simulink model "SunsensorActuatorsDrag"  (R2021b)
settings: Solver=FixedStepAuto  StartTime=0.0  StopTime=T  FixedStep=0.1  RelTol=1e-3
values from neighbouring files (symbols this model uses):
  a = 1/( 2/norm(r0) - dot(v0,v0)/mu_E )    [Excercise1_2223.m]    (also in Excercise2_2223.m; Lab08_script.m = 42164; Lab7_script.m = 16733.65; Lab7_scriptscalar.m = 16733.65)
  A0 = eye(3)    [Lab08_script.m]    (also in Lab7_script.m; Lab7_scriptscalar.m; Lab_GG.m)
  alpha = deg2rad(11.5)    [Lab08_script.m]
  Area_mb = diag([A1 A2 A3 A4 A5 A6])    [Lab08_script.m]    (also in Lab7_script.m)
  Area_sp = diag([A7 A8 A9 A10])    [Lab08_script.m]    (also in Lab7_script.m)
  around_boresight = deg2rad(dms2degrees([0,0,around_boresight]))    [Lab08_script.m]
  cross_boresight = deg2rad(dms2degrees([0,0,cross_boresight]))    [Lab08_script.m]
  e = horizonsresults(:,2)    [Ex3-5.m]    (also in Excercise1_2223.m = 1/mu_E*cross(v,h)-r./vecnorm(r,2,2); Lab08_script.m = 0; Lab7_script.m = 0.1976; Lab7_scriptscalar.m = 0.1976)
  epsilon = (vecnorm(v,2,2)).^2/2-mu_E./vecnorm(r,2,2)    [Excercise1_2223.m]    (also in Lab08_script.m = deg2rad(23.45); Lab7_script.m = deg2rad(23.45); Lab7_scriptscalar.m = deg2rad(23.45))
  H0 = ( g1_0^2 + g1_1^2 + h1_1^2 )^(1/2)    (= 3.0115258674e-05)    [Lab08_script.m]
  I = [Ix 0 0; 0 Iy 0; 0 0 Iz]    [Lab08_script.m]    (also in Lab7_script.m; Lab7_scriptscalar.m; Lab_GG.m)
  i = horizonsresults(:,3)    [Ex3-5.m]    (also in Lab08_script.m = deg2rad(0); Lab7_script.m = deg2rad(60); Lab7_scriptscalar.m = deg2rad(60); ex3_Lambert.m = kep_arr_M(3))
  I_inv = inv(I)    [Lab08_script.m]    (also in Lab7_script.m; Lab7_scriptscalar.m; Lab_GG.m)
  i_matrix = [1 0 0; 0 cos(i) sin(i); 0 -sin(i) cos(i)]    [Lab08_script.m]
  m = [0.01; 0.05; 0.01]    [Lab08_script.m]
  mu_E = astroConstants(13)    [Chapter3.m]    (also in Ex3-5.m; Excercise1_2223.m; Excercise2_2223.m; Lab08_script.m)
  n = 10    [Chapter3.m]    (also in Lab08_script.m = sqrt(mu_E/(a^3)); Lab7_script.m = sqrt(mu_E/(a^3)); Lab7_scriptscalar.m = sqrt(mu_E/(a^3)); Lab_GG.m = sqrt(mu_E/( R_E+r_orbit)^3))
  n3 = [0;0;1]    [Lab08_script.m]    (also in Lab7_script.m; Lab7_scriptscalar.m)
  N_b_mb = [n1'; n2'; n3'; n4'; n5'; n6']    [Lab08_script.m]    (also in Lab7_script.m)
  N_b_sp = [n7'; n8'; n9'; n10']    [Lab08_script.m]    (also in Lab7_script.m)
  n_sun = 2*pi/T_sun    (= 1.99238499086e-07)    [Lab08_script.m]    (also in Lab7_script.m; Lab7_scriptscalar.m)
  P = Fe/c    (= 4.52666666667e-06)    [Lab08_script.m]    (also in Lab7_script.m; Lab7_scriptscalar.m)
  R_E = astroConstants(23)    [Lab08_script.m]    (also in Lab7_script.m; Lab7_scriptscalar.m; Lab_GG.m)
  r_mb = [base/2 0 0; 0 base/2 0; 0 0 height/2; -base/2 0 0; 0 -base/2 0; 0 0 -height/2]    [Lab08_script.m]
  r_sp = [0 length_p1/2+base/2 0; 0 length_p1/2+base/2 0; 0 -length_p2/2-base/2 0; 0 -length_p2/2-base/2 0]    [Lab08_script.m]
  rho_s_mb = 0.5    [Lab08_script.m]    (also in Lab7_script.m; Lab7_scriptscalar.m)
  rho_s_sp = 0.1    [Lab08_script.m]    (also in Lab7_script.m; Lab7_scriptscalar.m)
  Rs = astroConstants(2)    [Lab08_script.m]    (also in Lab7_script.m; Lab7_scriptscalar.m)
  theta0 = deg2rad(0)    [Lab08_script.m]    (also in Lab7_script.m = deg2rad(230); Lab7_scriptscalar.m = deg2rad(230))
  unit = [1 0 0]'    [Lab08_script.m]    (also in Lab_GG.m)
  v1 = [Y1(:,4) Y1(:,5) Y1(:,6)]    [Excercise2_2223.m]    (also in Lab08_script.m = [0 1 -1]'; Lab7_script.m = [0 1 -1]'; Lab7_scriptscalar.m = [0 1 -1]'; Lab_GG.m = [0 1 -1]')
  v2 = [Y2(:,4) Y2(:,5) Y2(:,6)]    [Excercise2_2223.m]    (also in Lab08_script.m = [-1 0 1]'; Lab7_script.m = [-1 0 1]'; Lab7_scriptscalar.m = [-1 0 1]'; Lab_GG.m = [-1 0 1]')
  v3 = [1 -1 0]'    [Lab08_script.m]    (also in Lab7_script.m; Lab7_scriptscalar.m; Lab_GG.m)
  w_0 = [wx_0 wy_0 wz_0]'    [Lab08_script.m]    (also in Lab7_script.m; Lab7_scriptscalar.m; Lab_GG.m)
  w_E = deg2rad(15.04/3600)    [Ex3-5.m]    (also in Lab08_script.m = deg2rad(15.04)/3600)
  wy_0 = 1e-06    [Lab08_script.m]    (also in Lab7_script.m; Lab7_scriptscalar.m; Lab_GG.m = 0)
undefined symbols (not defined in the file or in its folder): A_vect, Cd, h_N_target, L, m_N_unit, N_B_Matrix, weight
libraries: matrix_library x15, vrlib x13, dspmtrx3 x2, sharedutil x2, simulink_extras x1
(part 1 of 2)
settings Model: Creator=sferl  LastModifiedBy=Giovanni

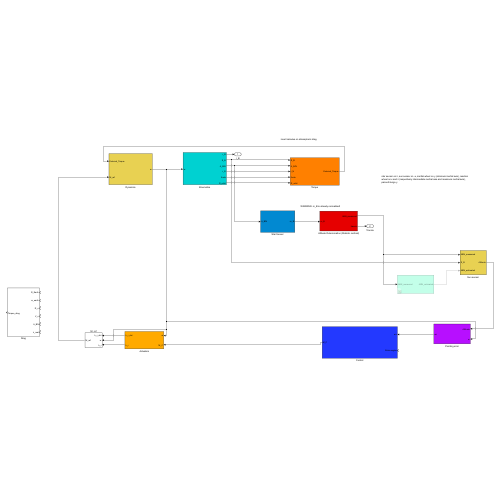
[thumbnail: Simulink's stored preview of the top-level diagram]
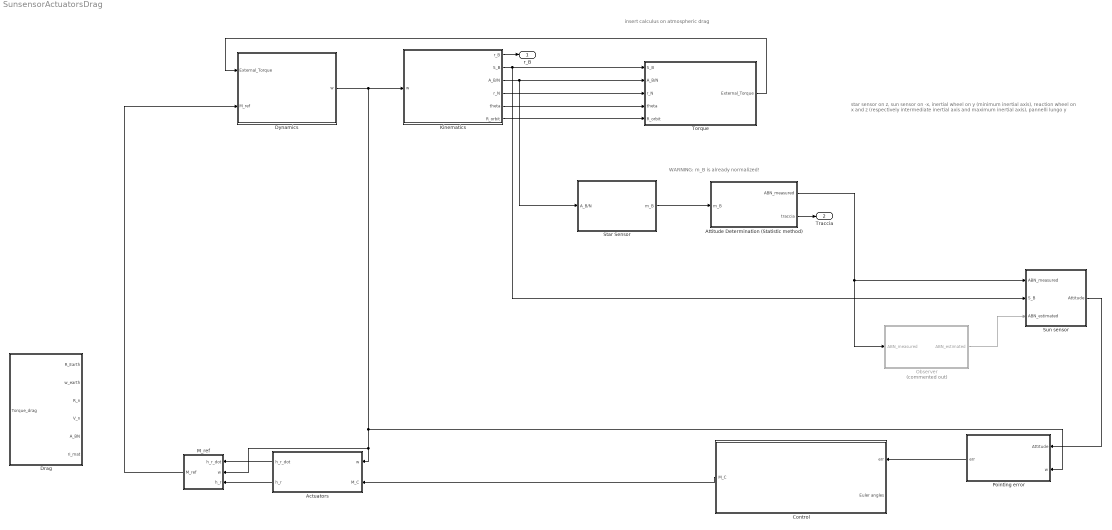
== system SunsensorActuatorsDrag ==
  note: insert calculus on atmospheric drag
  note: star sensor on z, sun sensor on -x, inertial wheel on y (minimum inertial axis), reaction wheel on x and z (respectively intermediate inertial axis and maximum inertial axis), pannelli lungo y
  note: WARNING: m_B is already normalized!
  Actuators : Subsystem
  Attitude Determination (Statistic method) : Subsystem
  Control : Subsystem
  Drag : Subsystem
  Dynamics : Subsystem
  Kinematics : Subsystem
  M_ref : Subsystem
  Observer : Subsystem  Commented=on
  Pointing error : Subsystem
  Star Sensor : Subsystem
  Sun sensor : Subsystem
  Torque : Subsystem
  r_B : Outport
  Traccia : Outport  Port=2
  wires:
  Kinematics/1(r_B) -> r_B/1
  Kinematics/3(A_B/N) -> Star Sensor/1(A_B/N), Torque/2(A_B/N)
  Star Sensor/1(m_B) -> Attitude Determination (Statistic method)/1(m_B)
  Kinematics/2(S_B) -> Sun sensor/2(S_B), Torque/1(S_B)
  Kinematics/4(r_N) -> Torque/3(r_N)
  Kinematics/5(theta) -> Torque/4(theta)
  Kinematics/6(R_orbit) -> Torque/5(R_orbit)
  Torque/1(External_Torque) -> Dynamics/1(External_Torque)
  Dynamics/1(w) -> Actuators/1(w), M_ref/2(w), Pointing error/2(w), Kinematics/1(w)
  Attitude Determination (Statistic method)/2(traccia) -> Traccia/1
  Pointing error/1(err) -> Control/1(err)
  Sun sensor/1(Attitude) -> Pointing error/1(Attitude)
  Attitude Determination (Statistic method)/1(ABN_measured) -> Sun sensor/1(ABN_measured), Observer/1(ABN_measured)
  Observer/1(ABN_estimated) -> Sun sensor/3(ABN_estimated)
  Control/1(M_C) -> Actuators/2(M_C)
  Actuators/1(h_r_dot) -> M_ref/1(h_r_dot)
  Actuators/2(h_r) -> M_ref/3(h_r)
  M_ref/1(M_ref) -> Dynamics/2(M_ref)

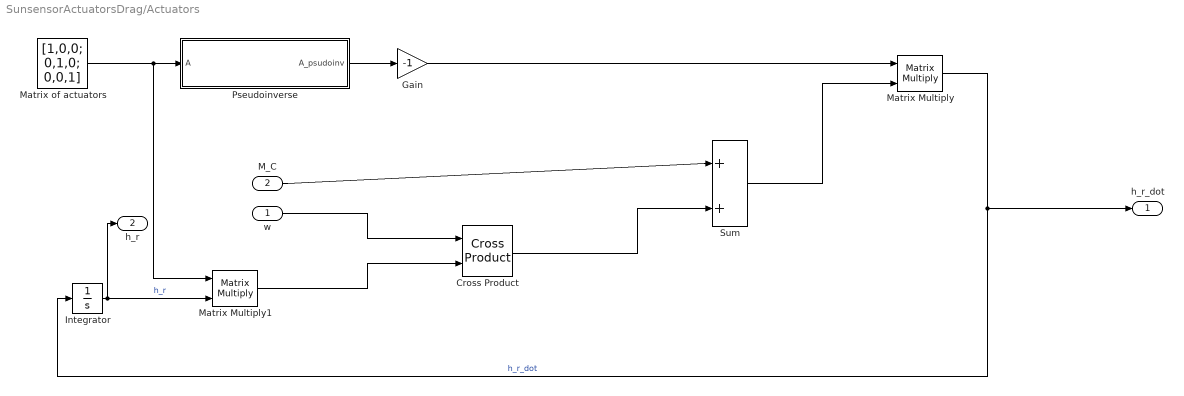
== system SunsensorActuatorsDrag/Actuators ==
  w : Inport
  M_C : Inport  Port=2
  Cross Product : matrix_library/Cross Product
  Gain : Gain  Gain=-1
  Integrator : Integrator  InitialCondition=[0; wy_0; 0]
  Matrix Multiply : Product  Multiplication=Matrix(*)
  Matrix Multiply1 : Product  Multiplication=Matrix(*)
  Matrix of actuators : Constant  Value=[1,0,0; 0,1,0; 0,0,1]
  Pseudoinverse : MATLAB Function  TreatAsAtomicUnit=on
  Sum : Sum  Inputs=|++
  h_r_dot : Outport
  h_r : Outport  Port=2
  wires:
  Matrix of actuators/1 -> Matrix Multiply1/1, Pseudoinverse/1(A)
  Pseudoinverse/1(A_psudoinv) -> Gain/1
  Gain/1 -> Matrix Multiply/1
  M_C/1 -> Sum/1
  w/1 -> Cross Product/1
  Matrix Multiply/1 -> h_r_dot/1, Integrator/1  "h_r_dot"
  Integrator/1 -> h_r/1, Matrix Multiply1/2  "h_r"
  Matrix Multiply1/1 -> Cross Product/2
  Cross Product/1 -> Sum/2
  Sum/1 -> Matrix Multiply/2

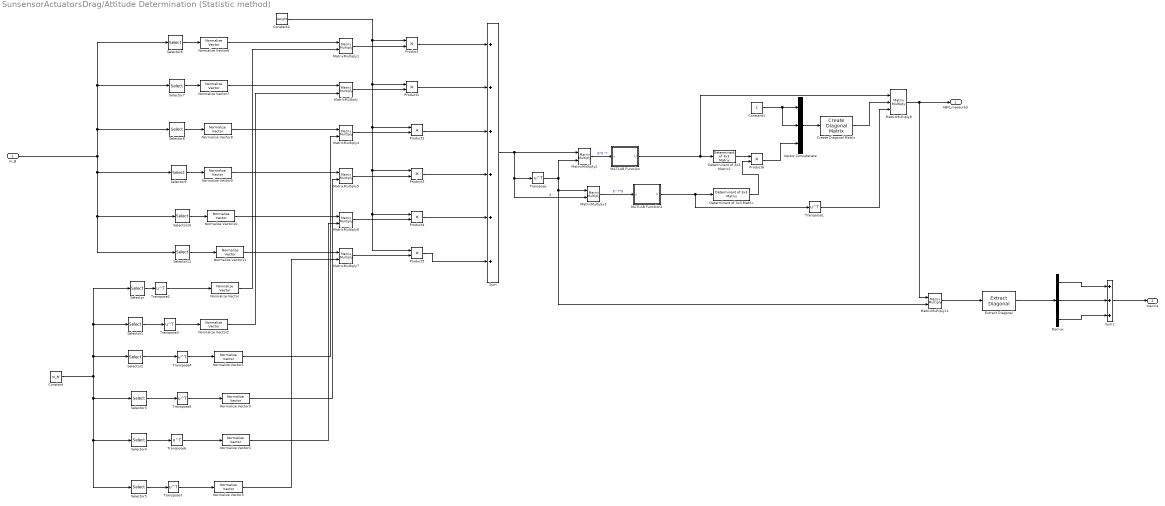
== system SunsensorActuatorsDrag/Attitude Determination (Statistic method) ==
  m_B : Inport
  Constant : Constant  Value=m_N'
  Constant1 : Constant
  Constant2 : Constant  Value=weight
  Create Diagonal Matrix : dspmtrx3/Create Diagonal Matrix
  Demux : Demux  Outputs=3
  Determinant of 3x3 Matrix : sharedutil/Determinant of 3x3 Matrix  aMode=aMode
  Determinant of 3x3 Matrix1 : sharedutil/Determinant of 3x3 Matrix  aMode=aMode
  Extract Diagonal : dspmtrx3/Extract Diagonal
  MATLAB Function : MATLAB Function  TreatAsAtomicUnit=on
  MATLAB Function1 : MATLAB Function  TreatAsAtomicUnit=on
  MatrixMultiply{,1..7,11} (9 alike) : Product  Multiplication=Matrix(*)
  MatrixMultiply8 : Product  Inputs=3  Multiplication=Matrix(*)
  Normalize Vector{,1..11} (12 alike) : vrlib/Utilities/Normalize Vector  maxzero=0
  Product{,1..6} (7 alike) : Product
  Selector : Selector  NumberOfDimensions=2  InputPortWidth=3  IndexOptions=Starting index (dialog),Starting index (dialog)  Indices=1,1  OutputSizes=3,1
  Selector1 : Selector  NumberOfDimensions=2  InputPortWidth=3  IndexOptions=Starting index (dialog),Starting index (dialog)  Indices=1,2  OutputSizes=3,1
  Selector10 : Selector  NumberOfDimensions=2  InputPortWidth=3  IndexOptions=Starting index (dialog),Starting index (dialog)  Indices=1,5  OutputSizes=3,1
  Selector11 : Selector  NumberOfDimensions=2  InputPortWidth=3  IndexOptions=Starting index (dialog),Starting index (dialog)  Indices=1,6  OutputSizes=3,1
  Selector2 : Selector  NumberOfDimensions=2  InputPortWidth=3  IndexOptions=Starting index (dialog),Starting index (dialog)  Indices=1,3  OutputSizes=3,1
  Selector3 : Selector  NumberOfDimensions=2  InputPortWidth=3  IndexOptions=Starting index (dialog),Starting index (dialog)  Indices=1,4  OutputSizes=3,1
  Selector4 : Selector  NumberOfDimensions=2  InputPortWidth=3  IndexOptions=Starting index (dialog),Starting index (dialog)  Indices=1,5  OutputSizes=3,1
  Selector5 : Selector  NumberOfDimensions=2  InputPortWidth=3  IndexOptions=Starting index (dialog),Starting index (dialog)  Indices=1,6  OutputSizes=3,1
  Selector6 : Selector  NumberOfDimensions=2  InputPortWidth=3  IndexOptions=Starting index (dialog),Starting index (dialog)  Indices=1,1  OutputSizes=3,1
  Selector7 : Selector  NumberOfDimensions=2  InputPortWidth=3  IndexOptions=Starting index (dialog),Starting index (dialog)  Indices=1,2  OutputSizes=3,1
  Selector8 : Selector  NumberOfDimensions=2  InputPortWidth=3  IndexOptions=Starting index (dialog),Starting index (dialog)  Indices=1,3  OutputSizes=3,1
  Selector9 : Selector  NumberOfDimensions=2  InputPortWidth=3  IndexOptions=Starting index (dialog),Starting index (dialog)  Indices=1,4  OutputSizes=3,1
  Sum : Sum  Inputs=++++++
  Sum1 : Sum  Inputs=+++
  Transpose{,1..7} (8 alike) : Math  Operator=transpose  SaturateOnIntegerOverflow=on
  Vector Concatenate : Concatenate  NumInputs=3
  ABN_measured : Outport
  traccia : Outport  Port=2
  wires:
  Transpose/1 -> MatrixMultiply11/2, MatrixMultiply3/1, MatrixMultiply2/2
  Constant2/1 -> Product3/1, Product4/1, Product5/1, Product2/1, Product1/1, Product/1
  Product2/1 -> Sum/3
  MatrixMultiply/1 -> Product1/2
  Product1/1 -> Sum/2
  MatrixMultiply7/1 -> Product5/2
  Sum/1 -> MatrixMultiply3/2, Transpose/1, MatrixMultiply2/1  "B"
  MatrixMultiply2/1 -> MATLAB Function/1(u)  "B*B^T"
  Product5/1 -> Sum/6
  MatrixMultiply5/1 -> Product3/2
  Product4/1 -> Sum/5
  Product/1 -> Sum/1
  MatrixMultiply4/1 -> Product2/2
  MatrixMultiply1/1 -> Product/2
  Product3/1 -> Sum/4
  MatrixMultiply6/1 -> Product4/2
  Selector1/1 -> Transpose3/1
  Selector3/1 -> Transpose5/1
  Selector4/1 -> Transpose6/1
  Constant/1 -> Selector3/1, Selector4/1, Selector5/1, Selector/1, Selector1/1, Selector2/1
  Selector2/1 -> Transpose4/1
  Selector5/1 -> Transpose7/1
  m_B/1 -> Selector6/1, Selector7/1, Selector8/1, Selector11/1, Selector10/1, Selector9/1
  Determinant of 3x3 Matrix1/1 -> Product6/1
  Determinant of 3x3 Matrix/1 -> Product6/2
  Constant1/1 -> Vector Concatenate/2, Vector Concatenate/1
  Product6/1 -> Vector Concatenate/3
  Vector Concatenate/1 -> Create Diagonal Matrix/1
  Create Diagonal Matrix/1 -> MatrixMultiply8/2
  MATLAB Function/1(U) -> MatrixMultiply8/1, Determinant of 3x3 Matrix1/1
  Transpose1/1 -> MatrixMultiply8/3
  MatrixMultiply8/1 -> MatrixMultiply11/1, ABN_measured/1
  MatrixMultiply3/1 -> MATLAB Function1/1(u)  "B^T*B"
  MATLAB Function1/1(V) -> Transpose1/1, Determinant of 3x3 Matrix/1
  MatrixMultiply11/1 -> Extract Diagonal/1
  Extract Diagonal/1 -> Demux/1
  Demux/1 -> Sum1/1
  Demux/2 -> Sum1/2
  Demux/3 -> Sum1/3
  Sum1/1 -> traccia/1
  Selector6/1 -> Normalize Vector6/1
  Selector7/1 -> Normalize Vector7/1
  Selector8/1 -> Normalize Vector8/1
  Selector9/1 -> Normalize Vector9/1
  Selector10/1 -> Normalize Vector10/1
  Selector11/1 -> Normalize Vector11/1
  Selector/1 -> Transpose2/1
  Transpose3/1 -> Normalize Vector2/1
  Transpose2/1 -> Normalize Vector/1
  Transpose4/1 -> Normalize Vector1/1
  Transpose5/1 -> Normalize Vector3/1
  Transpose6/1 -> Normalize Vector4/1
  Transpose7/1 -> Normalize Vector5/1
  Normalize Vector/1 -> MatrixMultiply1/2
  Normalize Vector2/1 -> MatrixMultiply/2
  Normalize Vector1/1 -> MatrixMultiply4/2
  Normalize Vector3/1 -> MatrixMultiply5/2
  Normalize Vector4/1 -> MatrixMultiply6/2
  Normalize Vector5/1 -> MatrixMultiply7/2
  Normalize Vector6/1 -> MatrixMultiply1/1
  Normalize Vector7/1 -> MatrixMultiply/1
  Normalize Vector8/1 -> MatrixMultiply4/1
  Normalize Vector9/1 -> MatrixMultiply5/1
  Normalize Vector10/1 -> MatrixMultiply6/1
  Normalize Vector11/1 -> MatrixMultiply7/1

== system SunsensorActuatorsDrag/Control ==
  note: potrei anche usare A e B al posto di SYS
  note: costruisci matrice controllo secondo slide 3 pacchetto 13b per ottenere stati
  err : Inport
  Euler angles : Inport  Port=2
  Gain : Gain  Gain=-1
  MATLAB Function : MATLAB Function  TreatAsAtomicUnit=on
  Matrix Multiply : Product  Multiplication=Matrix(*)
  M_C : Outport
  wires:
  err/1 -> Matrix Multiply/1
  Euler angles/1 -> ?
  MATLAB Function/1(K) -> Gain/1
  Gain/1 -> Matrix Multiply/2
  Matrix Multiply/1 -> M_C/1

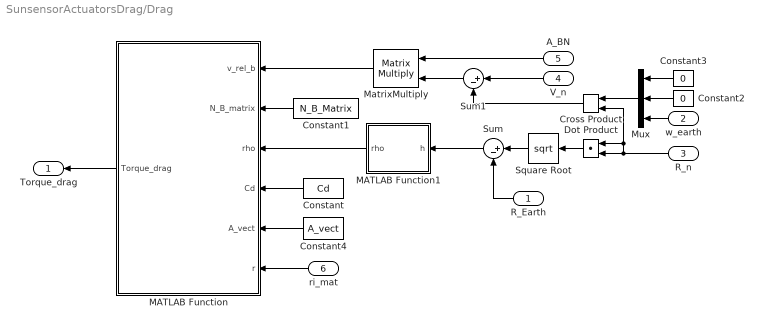
== system SunsensorActuatorsDrag/Drag ==
  R_Earth : Inport
  w_earth : Inport  Port=2
  R_n : Inport  Port=3
  V_n : Inport  Port=4
  A_BN : Inport  Port=5
  ri_mat : Inport  Port=6
  Constant : Constant  Value=Cd
  Constant1 : Constant  Value=N_B_Matrix
  Constant2 : Constant  Value=0
  Constant3 : Constant  Value=0
  Constant4 : Constant  Value=A_vect
  Cross Product : vrlib/Utilities/Cross Product
  Dot Product : DotProduct  InputSameDT=on  OutDataTypeStr=Inherit: Inherit via internal rule
  MATLAB Function : MATLAB Function  TreatAsAtomicUnit=on
  MATLAB Function1 : MATLAB Function  TreatAsAtomicUnit=on
  MatrixMultiply : Product  Multiplication=Matrix(*)
  Mux : Mux  Inputs=3
  Square Root : Sqrt  SaturateOnIntegerOverflow=on
  Sum : Sum  Inputs=|+-
  Sum1 : Sum  Inputs=|+-
  Torque_drag : Outport
  wires:
  MATLAB Function1/1(rho) -> MATLAB Function/3(rho)
  R_n/1 -> Cross Product/2, Dot Product/1, Dot Product/2
  Dot Product/1 -> Square Root/1
  Square Root/1 -> Sum/1
  R_Earth/1 -> Sum/2
  Sum/1 -> MATLAB Function1/1(h)
  MATLAB Function/1(Torque_drag) -> Torque_drag/1
  Constant/1 -> MATLAB Function/4(Cd)
  Constant1/1 -> MATLAB Function/2(N_B_matrix)
  Constant2/1 -> Mux/2
  Constant3/1 -> Mux/1
  w_earth/1 -> Mux/3
  Mux/1 -> Cross Product/1
  Cross Product/1 -> Sum1/2
  V_n/1 -> Sum1/1
  A_BN/1 -> MatrixMultiply/1
  Sum1/1 -> MatrixMultiply/2
  MatrixMultiply/1 -> MATLAB Function/1(v_rel_b)
  Constant4/1 -> MATLAB Function/5(A_vect)
  ri_mat/1 -> MATLAB Function/6(r)

== system SunsensorActuatorsDrag/Dynamics ==
  External_Torque : Inport
  M_ref : Inport  Port=2
  Constant : Constant  Value=I  VectorParams1D=off
  Constant1 : Constant  Value=I_inv  VectorParams1D=off
  Cross Product : matrix_library/Cross Product
  Integrator : Integrator  InitialCondition=w_0
  Product : Product  Multiplication=Matrix(*)
  Product1 : Product  Multiplication=Matrix(*)
  Sum : Sum  Inputs=|++
  Sum1 : Sum  Inputs=|++
  w : Outport
  wires:
  Product/1 -> Cross Product/1
  Constant/1 -> Product/1
  Constant1/1 -> Product1/1
  Integrator/1 -> Cross Product/2, Product/2, w/1  "w"
  Product1/1 -> Integrator/1  "w_dot"
  Cross Product/1 -> Sum/2
  Sum/1 -> Product1/2
  External_Torque/1 -> Sum1/1
  M_ref/1 -> Sum1/2
  Sum1/1 -> Sum/1

== system SunsensorActuatorsDrag/Kinematics ==
  w : Inport
  Sun direction with respect to body frame (already normalized!) : Subsystem
  "radius of orbit in body frame and transformation matrix from inertial frame to body frame " : Subsystem
  r_B : Outport
  S_B : Outport  Port=2
  A_B/N : Outport  Port=3
  r_N : Outport  Port=4
  theta : Outport  Port=5
  R_orbit : Outport  Port=6
  wires:
  "radius of orbit in body frame and transformation matrix from inertial frame to body frame "/2(A_B/N) -> Sun direction with respect to body frame (already normalized!)/1(A_B/N), A_B/N/1
  "radius of orbit in body frame and transformation matrix from inertial frame to body frame "/1(r_B) -> r_B/1
  w/1 -> "radius of orbit in body frame and transformation matrix from inertial frame to body frame "/1(w)
  Sun direction with respect to body frame (already normalized!)/1(S_B) -> S_B/1
  "radius of orbit in body frame and transformation matrix from inertial frame to body frame "/3(r_N) -> r_N/1
  "radius of orbit in body frame and transformation matrix from inertial frame to body frame "/4(theta) -> theta/1
  "radius of orbit in body frame and transformation matrix from inertial frame to body frame "/5(R_orbit) -> R_orbit/1

== system SunsensorActuatorsDrag/M_ref ==
  h_r_dot : Inport
  w : Inport  Port=2
  h_r : Inport  Port=3
  A_act : Constant  Value=[1,0,0; 0,1,0; 0,0,1]
  A_act1 : Constant  Value=[1,0,0; 0,1,0; 0,0,1]
  Cross Product : matrix_library/Cross Product
  Gain : Gain  Gain=-1
  MatrixMultiply : Product  Multiplication=Matrix(*)
  MatrixMultiply1 : Product  Multiplication=Matrix(*)
  Sum : Sum  Inputs=|++
  M_ref : Outport
  wires:
  MatrixMultiply1/1 -> Cross Product/2
  MatrixMultiply/1 -> Sum/1
  Sum/1 -> Gain/1
  A_act/1 -> MatrixMultiply/1
  h_r_dot/1 -> MatrixMultiply/2
  Cross Product/1 -> Sum/2
  Gain/1 -> M_ref/1
  w/1 -> Cross Product/1
  A_act1/1 -> MatrixMultiply1/1
  h_r/1 -> MatrixMultiply1/2

== system SunsensorActuatorsDrag/Observer ==
  ABN_measured : Inport
  Integrator : Integrator
  matrix L : Constant  Value=L
  ABN_estimated : Outport
  wires:
  Integrator/1 -> ABN_estimated/1, Integrator/1
  matrix L/1 -> ?

== system SunsensorActuatorsDrag/Pointing error ==
  Attitude : Inport
  w : Inport  Port=2
  Angular momentum in body frame : Subsystem
  Pointing error : Subsystem
  angular momentum in inertial frame : Subsystem
  err : Outport
  wires:
  Angular momentum in body frame/1(h_B) -> angular momentum in inertial frame/2(h_B)
  w/1 -> Angular momentum in body frame/1(w)
  angular momentum in inertial frame/1(h_N) -> Pointing error/1(h_N)
  Attitude/1 -> angular momentum in inertial frame/1(A_B/N)
  Pointing error/1(err) -> err/1

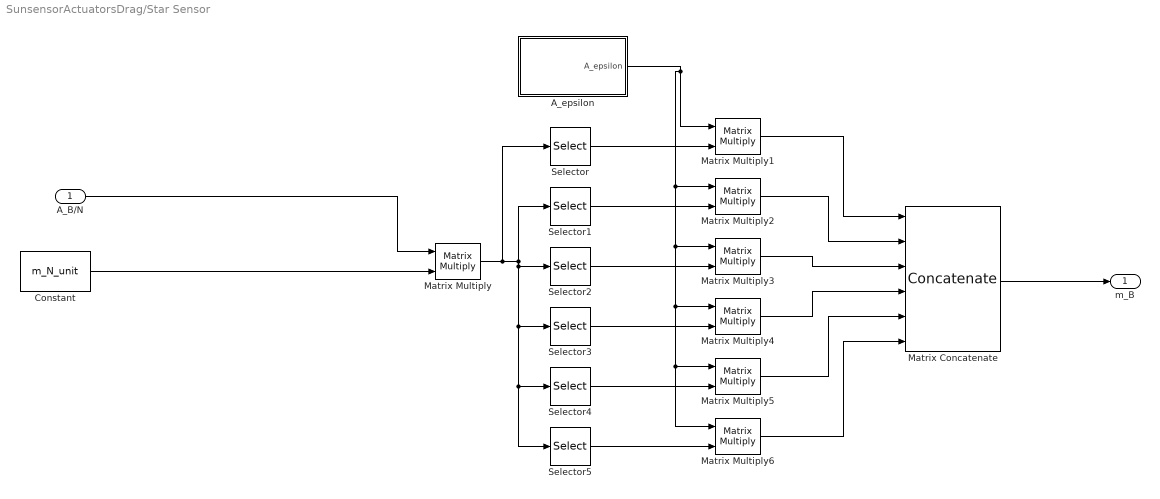
== system SunsensorActuatorsDrag/Star Sensor ==
  A_B/N : Inport
  A_epsilon : Subsystem
  Constant : Constant  Value=m_N_unit
  Matrix Concatenate : Concatenate  NumInputs=6  Mode=Multidimensional array  ConcatenateDimension=2
  Matrix Multiply{,1..6} (7 alike) : Product  Multiplication=Matrix(*)
  Selector : Selector  NumberOfDimensions=2  InputPortWidth=3  IndexOptions=Starting index (dialog),Starting index (dialog)  Indices=1,1  OutputSizes=3,1
  Selector1 : Selector  NumberOfDimensions=2  InputPortWidth=3  IndexOptions=Starting index (dialog),Starting index (dialog)  Indices=1,2  OutputSizes=3,1
  Selector2 : Selector  NumberOfDimensions=2  InputPortWidth=3  IndexOptions=Starting index (dialog),Starting index (dialog)  Indices=1,3  OutputSizes=3,1
  Selector3 : Selector  NumberOfDimensions=2  InputPortWidth=3  IndexOptions=Starting index (dialog),Starting index (dialog)  Indices=1,4  OutputSizes=3,1
  Selector4 : Selector  NumberOfDimensions=2  InputPortWidth=3  IndexOptions=Starting index (dialog),Starting index (dialog)  Indices=1,5  OutputSizes=3,1
  Selector5 : Selector  NumberOfDimensions=2  InputPortWidth=3  IndexOptions=Starting index (dialog),Starting index (dialog)  Indices=1,6  OutputSizes=3,1
  m_B : Outport
  wires:
  A_B/N/1 -> Matrix Multiply/1
  Constant/1 -> Matrix Multiply/2
  Matrix Multiply/1 -> Selector5/1, Selector4/1, Selector3/1, Selector2/1, Selector1/1, Selector/1
  A_epsilon/1(A_epsilon) -> Matrix Multiply6/1, Matrix Multiply5/1, Matrix Multiply4/1, Matrix Multiply3/1, Matrix Multiply2/1, Matrix Multiply1/1
  Selector/1 -> Matrix Multiply1/2
  Selector1/1 -> Matrix Multiply2/2
  Selector2/1 -> Matrix Multiply3/2
  Selector3/1 -> Matrix Multiply4/2
  Selector4/1 -> Matrix Multiply5/2
  Selector5/1 -> Matrix Multiply6/2
  Matrix Multiply1/1 -> Matrix Concatenate/1
  Matrix Multiply2/1 -> Matrix Concatenate/2
  Matrix Multiply3/1 -> Matrix Concatenate/3
  Matrix Multiply4/1 -> Matrix Concatenate/4
  Matrix Multiply5/1 -> Matrix Concatenate/5
  Matrix Multiply6/1 -> Matrix Concatenate/6
  Matrix Concatenate/1 -> m_B/1

== system SunsensorActuatorsDrag/Sun sensor ==
  note: if angle is <= 0.3, then the Sun is in (or in proximity of) the POV of the star sensor -> star sensor is turned off and I compute the new attitude starting from an estimation of the attitude relative to the latest measurements taken (see state observer block)
  note: if angle is > 0.3, then the Sun is not in (or in proximity of) the POV of the star sensor -> star sensor is turned on and I compute the attitude with its measurements (see attitude determination block)
  ABN_measured : Inport
  S_B : Inport  Port=2
  ABN_estimated : Inport  Port=3
  Acos : Trigonometry  Operator=acos
  Constant : Constant  Value=n3
  Matrix Multiply : Product
  Radians to Degrees : simulink_extras/Transformations/Radians to Degrees
  Switch : Switch  Criteria=u2 > Threshold  Threshold=0.3
  Attitude : Outport
  wires:
  S_B/1 -> Matrix Multiply/1
  Constant/1 -> Matrix Multiply/2
  Matrix Multiply/1 -> Acos/1  "cos(angle_between_n3_and_Sb)"
  ABN_measured/1 -> Switch/1
  ABN_estimated/1 -> Switch/3
  Switch/1 -> Attitude/1
  Acos/1 -> Radians to Degrees/1
  Radians to Degrees/1 -> Switch/2  "angle between S_B and n3 in degrees"

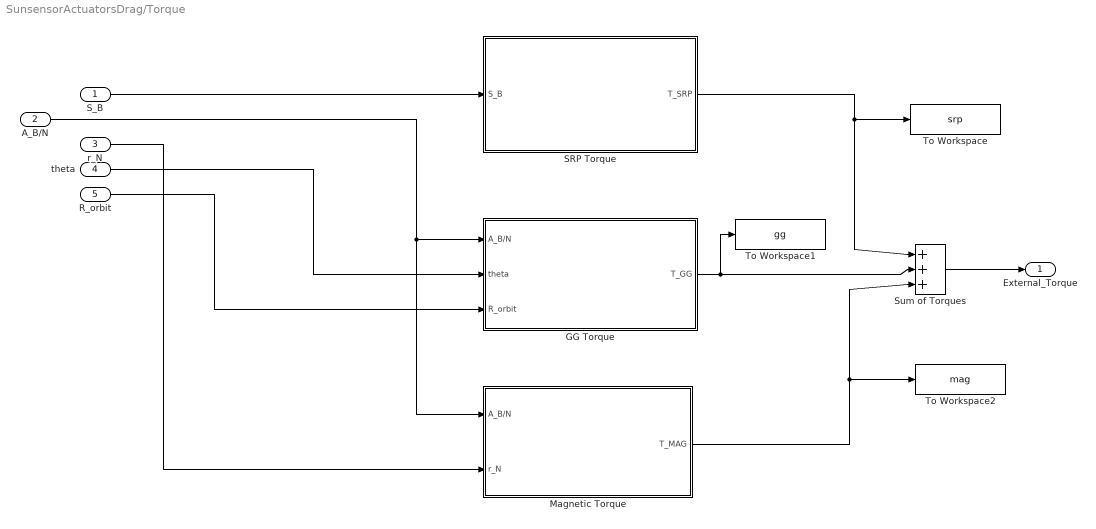
== system SunsensorActuatorsDrag/Torque ==
  S_B : Inport
  A_B/N : Inport  Port=2
  r_N : Inport  Port=3
  theta : Inport  Port=4
  R_orbit : Inport  Port=5
  GG Torque : Subsystem
  Magnetic Torque : Subsystem
  SRP Torque : Subsystem
  Sum of Torques : Sum  Inputs=+|+|+  CollapseMode=Specified dimension
  To Workspace : ToWorkspace  VariableName=srp  SampleTime=-1
  To Workspace1 : ToWorkspace  VariableName=gg  SampleTime=-1
  To Workspace2 : ToWorkspace  VariableName=mag  SampleTime=-1
  External_Torque : Outport
  wires:
  SRP Torque/1(T_SRP) -> To Workspace/1, Sum of Torques/1
  r_N/1 -> Magnetic Torque/2(r_N)
  GG Torque/1(T_GG) -> To Workspace1/1, Sum of Torques/2
  A_B/N/1 -> Magnetic Torque/1(A_B/N), GG Torque/1(A_B/N)
  R_orbit/1 -> GG Torque/3(R_orbit)
  Magnetic Torque/1(T_MAG) -> To Workspace2/1, Sum of Torques/3
  Sum of Torques/1 -> External_Torque/1
  S_B/1 -> SRP Torque/1(S_B)
  theta/1 -> GG Torque/2(theta)

== system SunsensorActuatorsDrag/Kinematics/Sun direction with respect to body frame (already normalized!) ==
  note: I divide the vector for its magnitude (Rs): this is the normalization!
  A_B/N : Inport
  Constant7 : Constant  Value=1/Rs
  MatrixMultiply : Product  Multiplication=Matrix(*)
  Product5 : Product
  S_N : Subsystem
  S_B : Outport
  wires:
  S_N/1(Out1) -> MatrixMultiply/2
  A_B/N/1 -> MatrixMultiply/1
  Constant7/1 -> Product5/1
  MatrixMultiply/1 -> Product5/2
  Product5/1 -> S_B/1

== system SunsensorActuatorsDrag/Kinematics/radius of orbit in body frame and transformation matrix from inertial frame to body frame  ==
  w : Inport
  MatrixMultiply1 : Product  Multiplication=Matrix(*)
  finder of A_B/N(t) : Subsystem
  orthonormalization of matrix A(t) : Subsystem
  radius of orbit in the inertial reference frame : Subsystem
  r_B : Outport
  A_B/N : Outport  Port=2
  r_N : Outport  Port=3
  theta : Outport  Port=4
  R_orbit : Outport  Port=5
  wires:
  finder of A_B/N(t)/1(A(t)) -> orthonormalization of matrix A(t)/1(A(t))
  orthonormalization of matrix A(t)/1(A_orthonorm) -> A_B/N/1, MatrixMultiply1/2
  MatrixMultiply1/1 -> r_B/1
  radius of orbit in the inertial reference frame/2(r_N) -> MatrixMultiply1/1, r_N/1
  w/1 -> finder of A_B/N(t)/1(w)
  radius of orbit in the inertial reference frame/1(theta) -> theta/1
  radius of orbit in the inertial reference frame/3(R_orbit) -> R_orbit/1

== system SunsensorActuatorsDrag/Pointing error/Angular momentum in body frame ==
  w : Inport
  Constant1 : Constant  Value=I
  Matrix Multiply : Product  Multiplication=Matrix(*)
  h_B : Outport
  wires:
  w/1 -> Matrix Multiply/2
  Matrix Multiply/1 -> h_B/1
  Constant1/1 -> Matrix Multiply/1

== system SunsensorActuatorsDrag/Pointing error/Pointing error ==
  h_N : Inport
  Abs : Abs
  Constant : Constant  Value=h_N_target  VectorParams1D=off
  Sum : Sum  Inputs=+-
  err : Outport
  wires:
  Constant/1 -> Sum/2
  h_N/1 -> Sum/1
  Sum/1 -> Abs/1
  Abs/1 -> err/1

== system SunsensorActuatorsDrag/Pointing error/angular momentum in inertial frame ==
  A_B/N : Inport
  h_B : Inport  Port=2
  Matrix Multiply : Product  Multiplication=Matrix(*)
  Transpose : Math  Operator=transpose  SaturateOnIntegerOverflow=on
  h_N : Outport
  wires:
  Transpose/1 -> Matrix Multiply/1
  Matrix Multiply/1 -> h_N/1
  A_B/N/1 -> Transpose/1
  h_B/1 -> Matrix Multiply/2

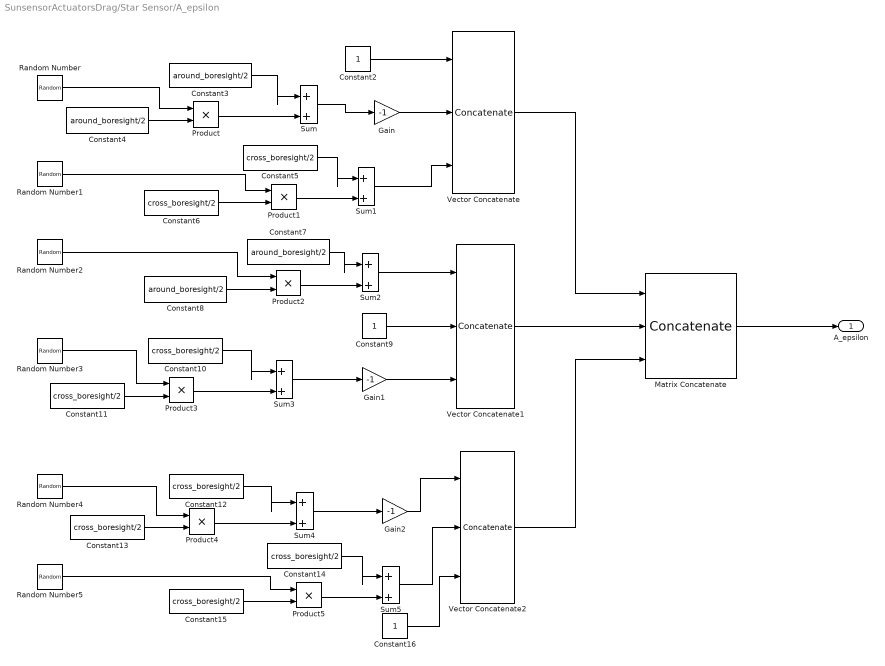
== system SunsensorActuatorsDrag/Star Sensor/A_epsilon ==
  Constant{5..6,10..15} (8 alike) : Constant  Value=cross_boresight/2
  Constant16 : Constant
  Constant2 : Constant
  Constant{3..4,7..8} (4 alike) : Constant  Value=around_boresight/2
  Constant9 : Constant
  Gain : Gain  Gain=-1
  Gain1 : Gain  Gain=-1
  Gain2 : Gain  Gain=-1
  Matrix Concatenate : Concatenate  NumInputs=3  Mode=Multidimensional array  ConcatenateDimension=2
  Product{,1..5} (6 alike) : Product
  Random Number{,1..5} (6 alike) : RandomNumber  Variance=0.16  SampleTime=0.1
  Sum{,1..5} (6 alike) : Sum  Inputs=|++
  Vector Concatenate : Concatenate  NumInputs=3  Mode=Multidimensional array
  Vector Concatenate1 : Concatenate  NumInputs=3  Mode=Multidimensional array
  Vector Concatenate2 : Concatenate  NumInputs=3  Mode=Multidimensional array
  A_epsilon : Outport
  wires:
  Constant10/1 -> Sum3/1
  Random Number/1 -> Product/1
  Constant12/1 -> Sum4/1
  Vector Concatenate2/1 -> Matrix Concatenate/3
  Constant11/1 -> Product3/2
  Sum/1 -> Gain/1
  Vector Concatenate1/1 -> Matrix Concatenate/2
  Constant3/1 -> Sum/1
  Product1/1 -> Sum1/2
  Constant15/1 -> Product5/2
  Constant16/1 -> Vector Concatenate2/3
  Product5/1 -> Sum5/2
  Constant13/1 -> Product4/2
  Product3/1 -> Sum3/2
  Constant6/1 -> Product1/2
  Product2/1 -> Sum2/2
  Constant7/1 -> Sum2/1
  Constant4/1 -> Product/2
  Constant9/1 -> Vector Concatenate1/2
  Constant8/1 -> Product2/2
  Sum2/1 -> Vector Concatenate1/1
  Gain/1 -> Vector Concatenate/2
  Sum3/1 -> Gain1/1
  Product4/1 -> Sum4/2
  Constant2/1 -> Vector Concatenate/1
  Sum5/1 -> Vector Concatenate2/2
  Vector Concatenate/1 -> Matrix Concatenate/1
  Product/1 -> Sum/2
  Sum1/1 -> Vector Concatenate/3
  Constant14/1 -> Sum5/1
  Gain1/1 -> Vector Concatenate1/3
  Gain2/1 -> Vector Concatenate2/1
  Constant5/1 -> Sum1/1
  Sum4/1 -> Gain2/1
  Matrix Concatenate/1 -> A_epsilon/1
  Random Number1/1 -> Product1/1
  Random Number2/1 -> Product2/1
  Random Number3/1 -> Product3/1
  Random Number4/1 -> Product4/1
  Random Number5/1 -> Product5/1

== system SunsensorActuatorsDrag/Torque/GG Torque ==
  A_B/N : Inport
  theta : Inport  Port=2
  R_orbit : Inport  Port=3
  Gravity Gradient : Subsystem
  Transformation from A_B/N to A_B/L : Subsystem
  T_GG : Outport
  wires:
  Gravity Gradient/1(T_GG) -> T_GG/1
  Transformation from A_B/N to A_B/L/1(A_B/L) -> Gravity Gradient/1(A_BL)
  A_B/N/1 -> Transformation from A_B/N to A_B/L/1(A_B/N)
  theta/1 -> Transformation from A_B/N to A_B/L/2(theta)
  R_orbit/1 -> Gravity Gradient/2(R_orbit)

== system SunsensorActuatorsDrag/Torque/Magnetic Torque ==
  A_B/N : Inport
  r_N : Inport  Port=2
  Cross Product : matrix_library/Cross Product
  magnetic field of Earth (modelled as dipole) in body frame : Subsystem
  parasitic magnetic torque : Constant  Value=m
  T_MAG : Outport
  wires:
  A_B/N/1 -> magnetic field of Earth (modelled as dipole) in body frame/1(A_B/N)
  magnetic field of Earth (modelled as dipole) in body frame/1(b_B) -> Cross Product/2
  parasitic magnetic torque/1 -> Cross Product/1
  Cross Product/1 -> T_MAG/1
  r_N/1 -> magnetic field of Earth (modelled as dipole) in body frame/2(r_N)

== system SunsensorActuatorsDrag/Torque/SRP Torque ==
  S_B : Inport
  Matrix Concatenate : Concatenate  Mode=Multidimensional array
  SRP Force on spacecraft main body : Subsystem
  SRP Force on spacecraft solar panels : Subsystem
  SRP Torque on spacecraft main body : Subsystem
  SRP Torque on spacecraft solar panels : Subsystem
  Sum of Elements : Sum  Inputs=+  CollapseMode=Specified dimension
  Transpose : Math  Operator=transpose  SaturateOnIntegerOverflow=on
  T_SRP : Outport
  wires:
  S_B/1 -> SRP Force on spacecraft main body/1(S_B), SRP Force on spacecraft solar panels/1(S_B)
  SRP Force on spacecraft solar panels/1(F_sp) -> SRP Torque on spacecraft solar panels/1(F_sp)
  SRP Force on spacecraft main body/1(F_mb) -> SRP Torque on spacecraft main body/1(F_mb)
  SRP Torque on spacecraft solar panels/1(T_sp) -> Matrix Concatenate/2
  SRP Torque on spacecraft main body/1(T_mb) -> Matrix Concatenate/1
  Sum of Elements/1 -> Transpose/1
  Transpose/1 -> T_SRP/1
  Matrix Concatenate/1 -> Sum of Elements/1

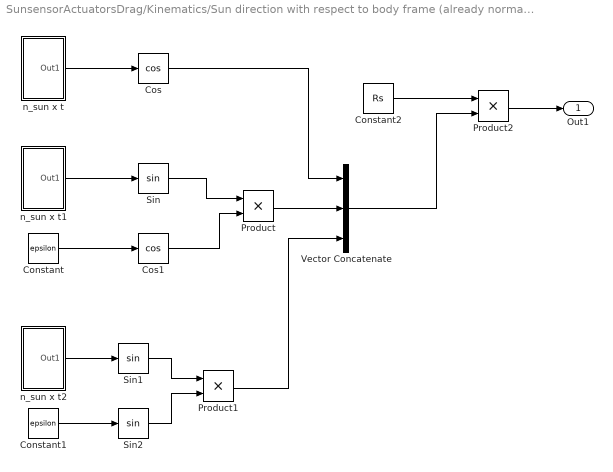
== system SunsensorActuatorsDrag/Kinematics/Sun direction with respect to body frame (already normalized!)/S_N ==
  Constant : Constant  Value=epsilon
  Constant1 : Constant  Value=epsilon
  Constant2 : Constant  Value=Rs
  Cos : Trigonometry  Operator=cos
  Cos1 : Trigonometry  Operator=cos
  Product : Product
  Product1 : Product
  Product2 : Product
  Sin : Trigonometry
  Sin1 : Trigonometry
  Sin2 : Trigonometry
  Vector Concatenate : Concatenate  NumInputs=3
  n_sun x t : Subsystem
  n_sun x t1 : Subsystem
  n_sun x t2 : Subsystem
  Out1 : Outport
  wires:
  n_sun x t2/1(Out1) -> Sin1/1
  Vector Concatenate/1 -> Product2/2
  Sin2/1 -> Product1/2
  Sin/1 -> Product/1
  n_sun x t1/1(Out1) -> Sin/1
  Product1/1 -> Vector Concatenate/3
  Constant2/1 -> Product2/1
  Cos/1 -> Vector Concatenate/1
  Cos1/1 -> Product/2
  Product/1 -> Vector Concatenate/2
  n_sun x t/1(Out1) -> Cos/1
  Constant1/1 -> Sin2/1
  Sin1/1 -> Product1/1
  Constant/1 -> Cos1/1
  Product2/1 -> Out1/1

== system SunsensorActuatorsDrag/Kinematics/radius of orbit in body frame and transformation matrix from inertial frame to body frame /finder of A_B//N(t) ==
  w : Inport
  Demux : Demux  Outputs=3
  Gain : Gain  Gain=-1
  Integrator1 : Integrator  InitialCondition=A0
  MatrixMultiply : Product  Multiplication=Matrix(*)
  w_hat : Subsystem
  A(t) : Outport
  wires:
  w/1 -> Demux/1
  Gain/1 -> MatrixMultiply/1
  Integrator1/1 -> A(t)/1, MatrixMultiply/2  "A(t)"
  w_hat/1(Out1) -> Gain/1
  Demux/3 -> w_hat/3(w_z)  "w_z"
  Demux/2 -> w_hat/2(w_y)  "w_y"
  Demux/1 -> w_hat/1(w_x)  "w_x"
  MatrixMultiply/1 -> Integrator1/1

== system SunsensorActuatorsDrag/Kinematics/radius of orbit in body frame and transformation matrix from inertial frame to body frame /orthonormalization of matrix A(t) ==
  A(t) : Inport
  Gain7 : Gain  Gain=3/2
  Gain8 : Gain  Gain=1/2
  MatrixMultiply3 : Product  Multiplication=Matrix(*)
  MatrixMultiply4 : Product  Multiplication=Matrix(*)
  Sum : Sum  Inputs=+-
  Transpose : Math  Operator=transpose  SaturateOnIntegerOverflow=on
  A_orthonorm : Outport
  wires:
  Transpose/1 -> MatrixMultiply3/2
  MatrixMultiply4/1 -> Sum/2
  MatrixMultiply3/1 -> MatrixMultiply4/1
  Gain7/1 -> Sum/1
  Gain8/1 -> MatrixMultiply4/2  "A/2"
  A(t)/1 -> Gain8/1, Transpose/1, MatrixMultiply3/1, Gain7/1
  Sum/1 -> A_orthonorm/1  "A_orthonorm"

== system SunsensorActuatorsDrag/Kinematics/radius of orbit in body frame and transformation matrix from inertial frame to body frame /radius of orbit in the inertial reference frame ==
  Product2 : Product
  Radius of orbit : Subsystem
  Theta : Subsystem
  vector [cos(theta); sin(theta)cos(i); sin(theta)sin(i)] : Subsystem
  theta : Outport
  r_N : Outport  Port=2
  R_orbit : Outport  Port=3
  wires:
  Theta/1(theta) -> vector [cos(theta); sin(theta)cos(i); sin(theta)sin(i)]/1(In1), theta/1, Radius of orbit/1(theta)
  Radius of orbit/1(R_orbit) -> Product2/1, R_orbit/1
  Product2/1 -> r_N/1
  vector [cos(theta); sin(theta)cos(i); sin(theta)sin(i)]/1(Out1) -> Product2/2

== system SunsensorActuatorsDrag/Torque/GG Torque/Gravity Gradient ==
  A_BL : Inport
  R_orbit : Inport  Port=2
  Constant4 : Constant  Value=I
  Cross Product1 : matrix_library/Cross Product
  MatrixMultiply4 : Product  Multiplication=Matrix(*)
  Product : Product
  To Workspace : ToWorkspace  VariableName=c_vector  SampleTime=-1
  creation of coefficient 3*mu_E/(R^3) : Subsystem
  creation of vector c : Subsystem
  T_GG : Outport
  wires:
  Constant4/1 -> MatrixMultiply4/1
  MatrixMultiply4/1 -> Cross Product1/2
  Cross Product1/1 -> Product/2
  Product/1 -> T_GG/1
  creation of vector c/1(c) -> To Workspace/1, MatrixMultiply4/2, Cross Product1/1
  A_BL/1 -> creation of vector c/1(A_BL)
  R_orbit/1 -> creation of coefficient 3*mu_E/(R^3)/1(In1)
  creation of coefficient 3*mu_E/(R^3)/1(Out1) -> Product/1

== system SunsensorActuatorsDrag/Torque/GG Torque/Transformation from A_B//N to A_B//L ==
  A_B/N : Inport
  theta : Inport  Port=2
  Constant : Constant  Value=i_matrix
  Matrix Multiply : Product  Multiplication=Matrix(*)
  MatrixMultiply1 : Product  Multiplication=Matrix(*)
  Transpose : Math  Operator=transpose  SaturateOnIntegerOverflow=on
  creation of A L/N : Subsystem
  A_B/L : Outport
  wires:
  A_B/N/1 -> MatrixMultiply1/1
  Transpose/1 -> MatrixMultiply1/2
  MatrixMultiply1/1 -> A_B/L/1  "A_BL"
  creation of A L/N/1(A_L/N) -> Matrix Multiply/1
  Constant/1 -> Matrix Multiply/2
  Matrix Multiply/1 -> Transpose/1
  theta/1 -> creation of A L/N/1(theta)

== system SunsensorActuatorsDrag/Torque/Magnetic Torque/magnetic field of Earth (modelled as dipole) in body frame ==
  A_B/N : Inport
  r_N : Inport  Port=2
  Matrix Multiply : Product  Multiplication=Matrix(*)
  b_N : Subsystem
  b_B : Outport
  wires:
  b_N/1(b_N) -> Matrix Multiply/2
  r_N/1 -> b_N/1(r_N)
  A_B/N/1 -> Matrix Multiply/1
  Matrix Multiply/1 -> b_B/1

== system SunsensorActuatorsDrag/Torque/SRP Torque/SRP Force on spacecraft main body ==
  S_B : Inport
  (1-rho_s)*Sb : Subsystem
  (2*rho_s*cos(theta)+2/3*rho_d)*Nb : Subsystem
  -PA*cos(theta) : Subsystem
  MatrixMultiply3 : Product  Multiplication=Matrix(*)
  Sum2 : Sum  Inputs=|++
  Switch to compute only force of exposed surfaces : Subsystem  TreatAsAtomicUnit=on
  compiute angle between incoming radiation and surface : Subsystem
  F_mb : Outport
  wires:
  S_B/1 -> (1-rho_s)*Sb/1(In1), compiute angle between incoming radiation and surface/1(S_B)
  compiute angle between incoming radiation and surface/1(cos_theta_mb) -> Switch to compute only force of exposed surfaces/1(In1)
  -PA*cos(theta)/1(Out1) -> MatrixMultiply3/1
  Sum2/1 -> MatrixMultiply3/2
  (1-rho_s)*Sb/1(Out1) -> Sum2/1
  (2*rho_s*cos(theta)+2/3*rho_d)*Nb/1(Out1) -> Sum2/2
  MatrixMultiply3/1 -> F_mb/1
  Switch to compute only force of exposed surfaces/1(Out1) -> -PA*cos(theta)/1(Input), (2*rho_s*cos(theta)+2/3*rho_d)*Nb/1(In1)

== system SunsensorActuatorsDrag/Torque/SRP Torque/SRP Force on spacecraft solar panels ==
  S_B : Inport
  (1-rho_s)*Sb : Subsystem
  (2*rho_s*cos(theta)+2/3*rho_d)*Nb : Subsystem
  -PA*cos(theta) : Subsystem
  MatrixMultiply3 : Product  Multiplication=Matrix(*)
  Sum2 : Sum  Inputs=|++
  Switch to compute only force of exposed surfaces : Subsystem  TreatAsAtomicUnit=on
  compiute angle between incoming radiation and surface : Subsystem
  F_sp : Outport
  wires:
  S_B/1 -> (1-rho_s)*Sb/1(In1), compiute angle between incoming radiation and surface/1(S_B)
  compiute angle between incoming radiation and surface/1(cos_theta_sp) -> Switch to compute only force of exposed surfaces/1(In1)
  -PA*cos(theta)/1(Out1) -> MatrixMultiply3/1
  Sum2/1 -> MatrixMultiply3/2
  (1-rho_s)*Sb/1(Out1) -> Sum2/1
  (2*rho_s*cos(theta)+2/3*rho_d)*Nb/1(Out1) -> Sum2/2
  MatrixMultiply3/1 -> F_sp/1
  Switch to compute only force of exposed surfaces/1(Out1) -> (2*rho_s*cos(theta)+2/3*rho_d)*Nb/1(In1), -PA*cos(theta)/1(In1)

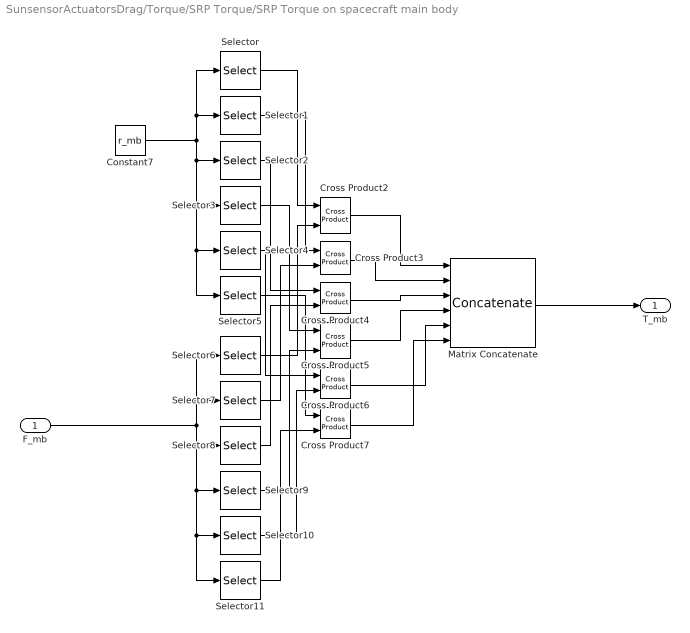
== system SunsensorActuatorsDrag/Torque/SRP Torque/SRP Torque on spacecraft main body ==
  F_mb : Inport
  Constant7 : Constant  Value=r_mb
  Cross Product{2..7} (6 alike) : matrix_library/Cross Product
  Matrix Concatenate : Concatenate  NumInputs=6  Mode=Multidimensional array
  Selector : Selector  NumberOfDimensions=2  InputPortWidth=3  IndexOptions=Starting index (dialog),Starting index (dialog)  Indices=1,1  OutputSizes=1,3
  Selector1 : Selector  NumberOfDimensions=2  InputPortWidth=3  IndexOptions=Starting index (dialog),Starting index (dialog)  Indices=2,1  OutputSizes=1,3
  Selector10 : Selector  NumberOfDimensions=2  InputPortWidth=3  IndexOptions=Starting index (dialog),Starting index (dialog)  Indices=5,1  OutputSizes=1,3
  Selector11 : Selector  NumberOfDimensions=2  InputPortWidth=3  IndexOptions=Starting index (dialog),Starting index (dialog)  Indices=6,1  OutputSizes=1,3
  Selector2 : Selector  NumberOfDimensions=2  InputPortWidth=3  IndexOptions=Starting index (dialog),Starting index (dialog)  Indices=3,1  OutputSizes=1,3
  Selector3 : Selector  NumberOfDimensions=2  InputPortWidth=3  IndexOptions=Starting index (dialog),Starting index (dialog)  Indices=4,1  OutputSizes=1,3
  Selector4 : Selector  NumberOfDimensions=2  InputPortWidth=3  IndexOptions=Starting index (dialog),Starting index (dialog)  Indices=5,1  OutputSizes=1,3
  Selector5 : Selector  NumberOfDimensions=2  InputPortWidth=3  IndexOptions=Starting index (dialog),Starting index (dialog)  Indices=6,1  OutputSizes=1,3
  Selector6 : Selector  NumberOfDimensions=2  InputPortWidth=3  IndexOptions=Starting index (dialog),Starting index (dialog)  Indices=1,1  OutputSizes=1,3
  Selector7 : Selector  NumberOfDimensions=2  InputPortWidth=3  IndexOptions=Starting index (dialog),Starting index (dialog)  Indices=2,1  OutputSizes=1,3
  Selector8 : Selector  NumberOfDimensions=2  InputPortWidth=3  IndexOptions=Starting index (dialog),Starting index (dialog)  Indices=3,1  OutputSizes=1,3
  Selector9 : Selector  NumberOfDimensions=2  InputPortWidth=3  IndexOptions=Starting index (dialog),Starting index (dialog)  Indices=4,1  OutputSizes=1,3
  T_mb : Outport
  wires:
  Constant7/1 -> Selector2/1, Selector5/1, Selector4/1, Selector3/1, Selector1/1, Selector/1
  Selector5/1 -> Cross Product7/1
  Selector10/1 -> Cross Product6/2
  Selector/1 -> Cross Product2/1
  F_mb/1 -> Selector8/1, Selector11/1, Selector10/1, Selector9/1, Selector7/1, Selector6/1
  Matrix Concatenate/1 -> T_mb/1
  Selector7/1 -> Cross Product3/2
  Cross Product3/1 -> Matrix Concatenate/2
  Selector2/1 -> Cross Product4/1
  Selector9/1 -> Cross Product5/2
  Cross Product6/1 -> Matrix Concatenate/5
  Selector6/1 -> Cross Product2/2
  Selector1/1 -> Cross Product3/1
  Cross Product2/1 -> Matrix Concatenate/1
  Selector11/1 -> Cross Product7/2
  Cross Product5/1 -> Matrix Concatenate/4
  Selector4/1 -> Cross Product6/1
  Selector3/1 -> Cross Product5/1
  Cross Product4/1 -> Matrix Concatenate/3
  Cross Product7/1 -> Matrix Concatenate/6
  Selector8/1 -> Cross Product4/2

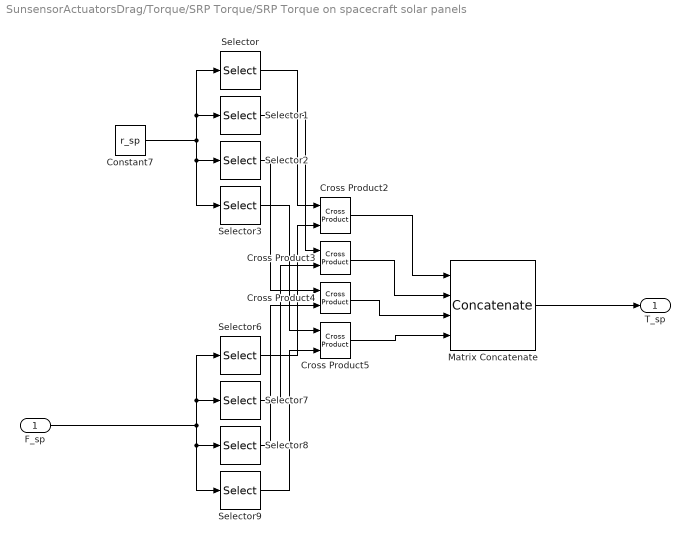
== system SunsensorActuatorsDrag/Torque/SRP Torque/SRP Torque on spacecraft solar panels ==
  F_sp : Inport
  Constant7 : Constant  Value=r_sp
  Cross Product{2..5} (4 alike) : matrix_library/Cross Product
  Matrix Concatenate : Concatenate  NumInputs=4  Mode=Multidimensional array
  Selector : Selector  NumberOfDimensions=2  InputPortWidth=3  IndexOptions=Starting index (dialog),Starting index (dialog)  Indices=1,1  OutputSizes=1,3
  Selector1 : Selector  NumberOfDimensions=2  InputPortWidth=3  IndexOptions=Starting index (dialog),Starting index (dialog)  Indices=2,1  OutputSizes=1,3
  Selector2 : Selector  NumberOfDimensions=2  InputPortWidth=3  IndexOptions=Starting index (dialog),Starting index (dialog)  Indices=3,1  OutputSizes=1,3
  Selector3 : Selector  NumberOfDimensions=2  InputPortWidth=3  IndexOptions=Starting index (dialog),Starting index (dialog)  Indices=4,1  OutputSizes=1,3
  Selector6 : Selector  NumberOfDimensions=2  InputPortWidth=3  IndexOptions=Starting index (dialog),Starting index (dialog)  Indices=1,1  OutputSizes=1,3
  Selector7 : Selector  NumberOfDimensions=2  InputPortWidth=3  IndexOptions=Starting index (dialog),Starting index (dialog)  Indices=2,1  OutputSizes=1,3
  Selector8 : Selector  NumberOfDimensions=2  InputPortWidth=3  IndexOptions=Starting index (dialog),Starting index (dialog)  Indices=3,1  OutputSizes=1,3
  Selector9 : Selector  NumberOfDimensions=2  InputPortWidth=3  IndexOptions=Starting index (dialog),Starting index (dialog)  Indices=4,1  OutputSizes=1,3
  T_sp : Outport
  wires:
  Constant7/1 -> Selector2/1, Selector3/1, Selector1/1, Selector/1
  Selector/1 -> Cross Product2/1
  F_sp/1 -> Selector8/1, Selector9/1, Selector7/1, Selector6/1
  Matrix Concatenate/1 -> T_sp/1
  Selector7/1 -> Cross Product3/2
  Cross Product3/1 -> Matrix Concatenate/2
  Selector2/1 -> Cross Product4/1
  Selector9/1 -> Cross Product5/2
  Selector6/1 -> Cross Product2/2
  Selector1/1 -> Cross Product3/1
  Cross Product2/1 -> Matrix Concatenate/1
  Cross Product5/1 -> Matrix Concatenate/4
  Selector3/1 -> Cross Product5/1
  Cross Product4/1 -> Matrix Concatenate/3
  Selector8/1 -> Cross Product4/2

== system SunsensorActuatorsDrag/Kinematics/Sun direction with respect to body frame (already normalized!)/S_N/n_sun x t ==
  Clock : Clock
  Constant : Constant  Value=n_sun
  Product : Product
  Out1 : Outport
  wires:
  Constant/1 -> Product/1
  Clock/1 -> Product/2
  Product/1 -> Out1/1

== system SunsensorActuatorsDrag/Kinematics/Sun direction with respect to body frame (already normalized!)/S_N/n_sun x t1 ==
  Clock : Clock
  Constant : Constant  Value=n_sun
  Product : Product
  Out1 : Outport
  wires:
  Product/1 -> Out1/1
  Clock/1 -> Product/2
  Constant/1 -> Product/1

== system SunsensorActuatorsDrag/Kinematics/Sun direction with respect to body frame (already normalized!)/S_N/n_sun x t2 ==
  Clock : Clock
  Constant : Constant  Value=n_sun
  Product : Product
  Out1 : Outport
  wires:
  Constant/1 -> Product/1
  Clock/1 -> Product/2
  Product/1 -> Out1/1

== system SunsensorActuatorsDrag/Kinematics/radius of orbit in body frame and transformation matrix from inertial frame to body frame /finder of A_B//N(t)/w_hat ==
  w_x : Inport
  w_y : Inport  Port=2
  w_z : Inport  Port=3
  Matrix Concatenate : Concatenate  NumInputs=3  Mode=Multidimensional array  ConcatenateDimension=2
  Scope : Scope  NumInputPorts=3
  Subsystem : Subsystem
  Subsystem1 : Subsystem
  Subsystem2 : Subsystem
  Out1 : Outport
  wires:
  w_y/1 -> Subsystem1/2(w_y), Subsystem/2(w_y), Subsystem2/2(w_y), Scope/2
  w_z/1 -> Subsystem2/3(w_z), Subsystem/3(w_z), Subsystem1/3(w_z), Scope/3
  w_x/1 -> Subsystem2/1(w_x), Subsystem/1(w_x), Subsystem1/1(w_x), Scope/1
  Subsystem2/1(Out1) -> Matrix Concatenate/3
  Subsystem1/1(Out1) -> Matrix Concatenate/2
  Subsystem/1(Out1) -> Matrix Concatenate/1
  Matrix Concatenate/1 -> Out1/1

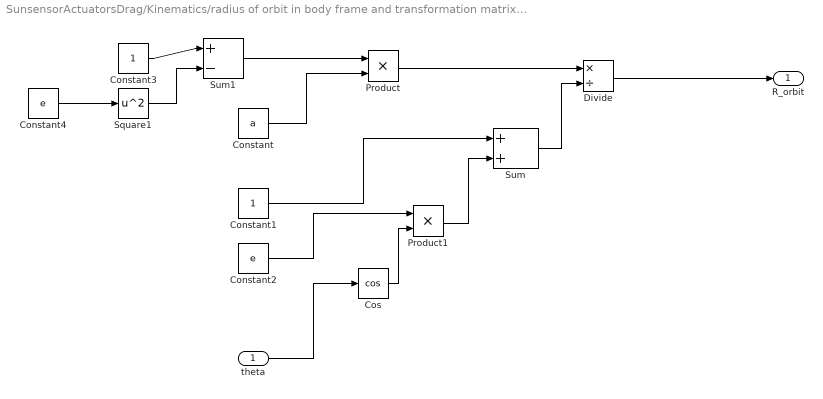
== system SunsensorActuatorsDrag/Kinematics/radius of orbit in body frame and transformation matrix from inertial frame to body frame /radius of orbit in the inertial reference frame/Radius of orbit ==
  theta : Inport
  Constant : Constant  Value=a
  Constant1 : Constant
  Constant2 : Constant  Value=e
  Constant3 : Constant
  Constant4 : Constant  Value=e
  Cos : Trigonometry  Operator=cos
  Divide : Product  Inputs=*/
  Product : Product
  Product1 : Product
  Square1 : Math  Operator=square  SaturateOnIntegerOverflow=on
  Sum : Sum  Inputs=|++
  Sum1 : Sum  Inputs=|+-
  R_orbit : Outport
  wires:
  Sum/1 -> Divide/2
  Constant1/1 -> Sum/1
  Square1/1 -> Sum1/2
  Product1/1 -> Sum/2
  Constant2/1 -> Product1/1
  Constant/1 -> Product/2
  Divide/1 -> R_orbit/1
  Cos/1 -> Product1/2
  Sum1/1 -> Product/1
  theta/1 -> Cos/1
  Constant4/1 -> Square1/1
  Constant3/1 -> Sum1/1
  Product/1 -> Divide/1

== system SunsensorActuatorsDrag/Kinematics/radius of orbit in body frame and transformation matrix from inertial frame to body frame /radius of orbit in the inertial reference frame/Theta ==
  Denominator : Subsystem
  Divide : Product  Inputs=*/
  Integrator : Integrator  InitialCondition=theta0
  Numerator : Subsystem
  theta : Outport
  wires:
  Numerator/1(Out1) -> Divide/1
  Denominator/1(Out1) -> Divide/2
  Integrator/1 -> theta/1, Numerator/1(In1)
  Divide/1 -> Integrator/1

== system SunsensorActuatorsDrag/Kinematics/radius of orbit in body frame and transformation matrix from inertial frame to body frame /radius of orbit in the inertial reference frame/vector [cos(theta); sin(theta)cos(i); sin(theta)sin(i)] ==
  In1 : Inport
  Constant : Constant  Value=i
  Constant1 : Constant  Value=i
  Cos : Trigonometry  Operator=cos
  Cos1 : Trigonometry  Operator=cos
  Product : Product
  Product1 : Product
  Sin : Trigonometry
  Sin1 : Trigonometry
  Sin2 : Trigonometry
  Vector Concatenate : Concatenate  NumInputs=3
  Out1 : Outport
  wires:
  Sin/1 -> Product/1
  Sin2/1 -> Product1/1
  Constant1/1 -> Sin1/1
  Cos/1 -> Vector Concatenate/1
  Product/1 -> Vector Concatenate/2
  In1/1 -> Sin2/1, Sin/1, Cos/1
  Constant/1 -> Cos1/1
  Cos1/1 -> Product/2
  Sin1/1 -> Product1/2
  Product1/1 -> Vector Concatenate/3
  Vector Concatenate/1 -> Out1/1

== system SunsensorActuatorsDrag/Torque/GG Torque/Gravity Gradient/creation of coefficient 3*mu_E//(R^3) ==
  In1 : Inport
  Constant : Constant  Value=3
  Constant1 : Constant  Value=mu_E
  Divide : Product  Inputs=*/
  Gain : Gain  Gain=3
  Power : Math  Operator=pow  SaturateOnIntegerOverflow=on
  Out1 : Outport
  wires:
  Divide/1 -> Out1/1
  Power/1 -> Divide/2
  Constant/1 -> Power/2
  In1/1 -> Power/1
  Constant1/1 -> Gain/1
  Gain/1 -> Divide/1

== system SunsensorActuatorsDrag/Torque/GG Torque/Gravity Gradient/creation of vector c ==
  A_BL : Inport
  Constant : Constant  Value=unit  VectorParams1D=off
  MatrixMultiply3 : Product  Multiplication=Matrix(*)
  c : Outport
  wires:
  A_BL/1 -> MatrixMultiply3/1
  MatrixMultiply3/1 -> c/1
  Constant/1 -> MatrixMultiply3/2

== system SunsensorActuatorsDrag/Torque/GG Torque/Transformation from A_B//N to A_B//L/creation of A L//N ==
  theta : Inport
  Matrix Concatenate : Concatenate  NumInputs=3  Mode=Multidimensional array  ConcatenateDimension=2
  first column of A_L/N : Subsystem
  second column of A_L/N : Subsystem
  third column of A_L/N : Subsystem
  A_L/N : Outport
  wires:
  second column of A_L/N/1(A_L/N (:,2)) -> Matrix Concatenate/2
  Matrix Concatenate/1 -> A_L/N/1
  first column of A_L/N/1(A_L/N (:,1)) -> Matrix Concatenate/1
  third column of A_L/N/1(A_L/N (:,3)) -> Matrix Concatenate/3
  theta/1 -> second column of A_L/N/1(theta), first column of A_L/N/1(theta)

== system SunsensorActuatorsDrag/Torque/Magnetic Torque/magnetic field of Earth (modelled as dipole) in body frame/b_N ==
  r_N : Inport
  Product : Product
  R^3*H0/(r^3) : Subsystem
  "[3*(m_unit*r_unit)*r_unit - m_unit)" : Subsystem
  magnetic unit vector of Earth : Subsystem
  normalization of r_N : Subsystem
  b_N : Outport
  wires:
  magnetic unit vector of Earth/1(Out1) -> "[3*(m_unit*r_unit)*r_unit - m_unit)"/1(m_unit)
  normalization of r_N/1(normalized r_N) -> "[3*(m_unit*r_unit)*r_unit - m_unit)"/2(normalized r_N)
  normalization of r_N/2(norm(r_N)) -> R^3*H0/(r^3)/1(normalized r_N)
  "[3*(m_unit*r_unit)*r_unit - m_unit)"/1(Out1) -> Product/1
  Product/1 -> b_N/1
  R^3*H0/(r^3)/1(coeff) -> Product/2
  r_N/1 -> normalization of r_N/1(r_N)

== system SunsensorActuatorsDrag/Torque/SRP Torque/SRP Force on spacecraft main body/(1-rho_s)*Sb ==
  In1 : Inport
  Constant2 : Constant
  Constant3 : Constant  Value=rho_s_mb
  Product1 : Product
  Sum : Sum  Inputs=+-
  Transpose1 : Math  Operator=transpose  SaturateOnIntegerOverflow=on
  Out1 : Outport
  wires:
  Constant2/1 -> Sum/1
  Sum/1 -> Product1/1
  Transpose1/1 -> Product1/2
  Product1/1 -> Out1/1
  Constant3/1 -> Sum/2
  In1/1 -> Transpose1/1

== system SunsensorActuatorsDrag/Torque/SRP Torque/SRP Force on spacecraft main body/(2*rho_s*cos(theta)+2//3*rho_d)*Nb ==
  In1 : Inport
  Constant1 : Constant  Value=rho_s_mb
  Constant2 : Constant  Value=ones(6,1)
  Constant4 : Constant  Value=rho_s_mb
  Constant6 : Constant  Value=N_b_mb
  Gain1 : Gain  Gain=2
  Gain2 : Gain  Gain=2/3
  MatrixMultiply2 : Product  Multiplication=Matrix(*)
  Product : Product
  Product2 : Product
  Sum1 : Sum  Inputs=|++
  Out1 : Outport
  wires:
  Gain2/1 -> Product/1
  Product/1 -> Sum1/1
  MatrixMultiply2/1 -> Out1/1
  Constant4/1 -> Gain1/1
  In1/1 -> Product2/2
  Constant6/1 -> MatrixMultiply2/2
  Gain1/1 -> Product2/1
  Product2/1 -> Sum1/2
  Sum1/1 -> MatrixMultiply2/1
  Constant1/1 -> Gain2/1
  Constant2/1 -> Product/2

== system SunsensorActuatorsDrag/Torque/SRP Torque/SRP Force on spacecraft main body/-PA*cos(theta) ==
  Input : Inport
  Constant1 : Constant  Value=Area_mb
  Gain : Gain  Gain=-P
  Matrix Multiply : Product  Multiplication=Matrix(*)
  Out1 : Outport
  wires:
  Matrix Multiply/1 -> Out1/1
  Gain/1 -> Matrix Multiply/1
  Constant1/1 -> Gain/1
  Input/1 -> Matrix Multiply/2

== system SunsensorActuatorsDrag/Torque/SRP Torque/SRP Force on spacecraft main body/Switch to compute only force of exposed surfaces ==
  In1 : Inport  Partition=on  PartitionDimension=1  PartitionWidth=1  PartitionOffset=0
  Constant : Constant  Value=0
  For Each : ForEach  DisableCoverage=on
  Switch : Switch  Criteria=u2 > Threshold
  Out1 : Outport  ConcatenationDimension=1
  wires:
  In1/1 -> Switch/1, Switch/2
  Constant/1 -> Switch/3
  Switch/1 -> Out1/1
